simulink model "PatchedConic"  (R2022b)
settings: Solver=ode4  StartTime=0.0  StopTime=simTime  FixedStep=dt  RelTol=1e-3
values from neighbouring files (symbols this model uses):
  dv1 = [0,0.730140014317,0]    [main.m]
  lunar_distance = 388000    [main.m]
  lunar_w = [0,0,2*pi / (27*24*3600)]    [main.m]
  lunar_wn = 2*pi / (27*24*3600)    (= 2.6934093395e-06)    [main.m]
  mu_earth = 398600    [main.m]
  mu_lunar = 4911.3    [main.m]
  r0_inj = [lunar_distance - lunar_SOI ,0,0]    [main.m]
  r0_trans = [ - R_earth - altitude , 0 , 0]    [main.m]
  T_inj = 167185    [main.m]
  T_trans = pi * sqrt( a_trans ^3 / mu_earth )    [main.m]
  v0_inj = [ 0 , sqrt( mu_earth * ( 2 / (lunar_distance - lunar_SOI ) - 1 / a_trans ) ) , 0]    [main.m]
  v0_trans = [ 0 , -sqrt( mu_earth * ( 2 / norm(r0_trans) - 1 / a_trans ) ) , 0 ]    [main.m]
  v_need = sqrt ( mu_lunar / ( R_lunar + Rmission ) )    [main.m]
libraries: matrix_library x1
settings Model: Creator=dongmin  LastModifiedBy=dongmin

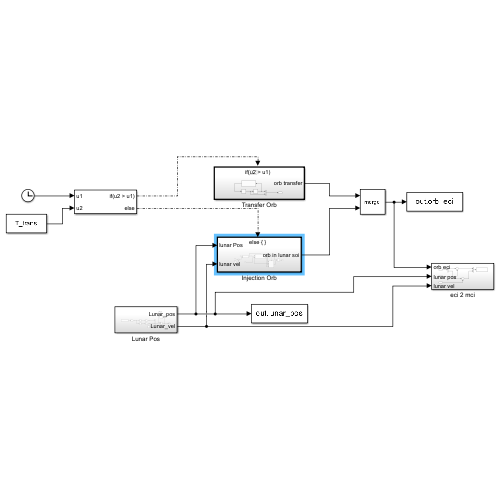
[thumbnail: Simulink's stored preview of the top-level diagram]
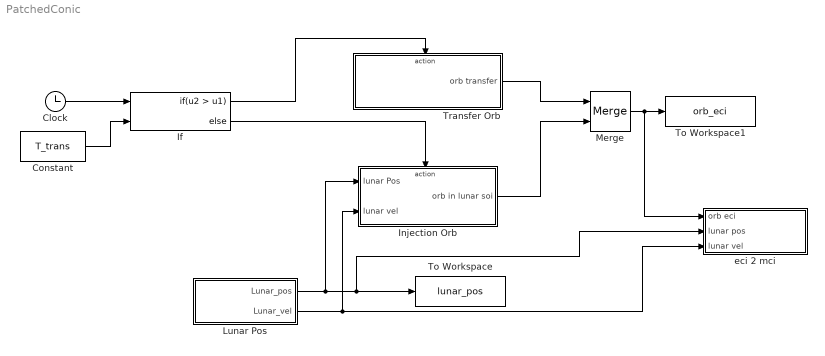
== system PatchedConic ==
  Clock : Clock
  Constant : Constant  Value=T_trans
  If : If  NumInputs=2  IfExpression=u2 > u1
  Injection Orb : Subsystem  TreatAsAtomicUnit=on
  Lunar Pos : Subsystem
  Merge : Merge
  To Workspace : ToWorkspace  VariableName=lunar_pos  SaveFormat=Timeseries  SampleTime=-1
  To Workspace1 : ToWorkspace  VariableName=orb_eci  SaveFormat=Timeseries  SampleTime=-1
  Transfer Orb : Subsystem  TreatAsAtomicUnit=on
  eci 2 mci : Subsystem
  wires:
  Clock/1 -> If/1
  Constant/1 -> If/2
  If/1 -> Transfer Orb/Action
  If/2 -> Injection Orb/Action
  Lunar Pos/1(Lunar_pos) -> Injection Orb/1(lunar Pos), eci 2 mci/2(lunar pos), To Workspace/1
  Transfer Orb/1(orb transfer) -> Merge/1
  Injection Orb/1(orb in lunar soi) -> Merge/2
  Merge/1 -> eci 2 mci/1(orb eci), To Workspace1/1
  Lunar Pos/2(Lunar_vel) -> Injection Orb/2(lunar vel), eci 2 mci/3(lunar vel)

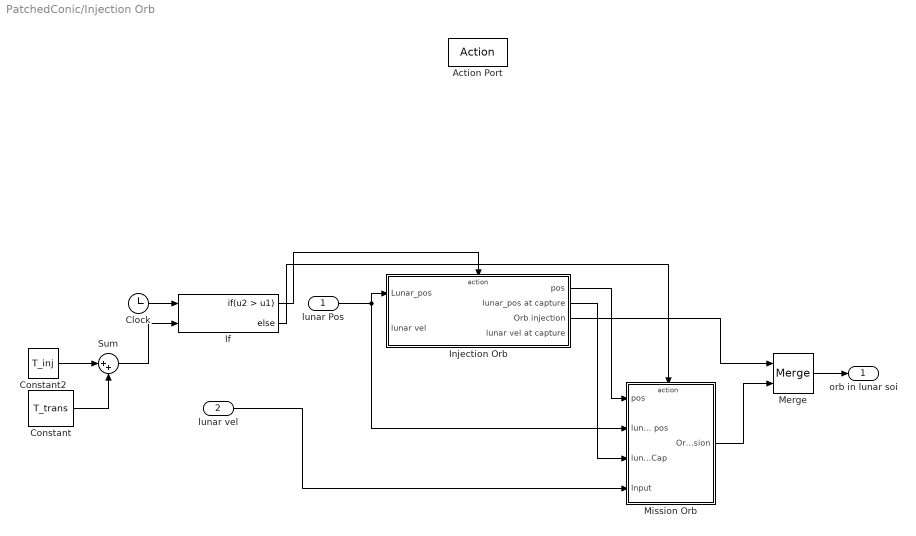
== system PatchedConic/Injection Orb ==
  lunar Pos : Inport
  lunar vel : Inport  Port=2
  Action Port : ActionPort  ActionPortLabel=else
  Clock : Clock
  Constant : Constant  Value=T_trans
  Constant2 : Constant  Value=T_inj
  If : If  NumInputs=2  IfExpression=u2 > u1
  Injection Orb : Subsystem  TreatAsAtomicUnit=on
  Merge : Merge
  Mission Orb : Subsystem  TreatAsAtomicUnit=on
  Sum : Sum  Inputs=|++
  orb in lunar soi : Outport
  wires:
  Clock/1 -> If/1
  Constant2/1 -> Sum/1
  If/1 -> Injection Orb/Action
  lunar Pos/1 -> Mission Orb/2(lunar pos), Injection Orb/1(Lunar_pos)
  If/2 -> Mission Orb/Action
  Injection Orb/1(pos) -> Mission Orb/1(pos)
  Constant/1 -> Sum/2
  Sum/1 -> If/2
  Injection Orb/2(lunar_pos at capture) -> Mission Orb/3(lunar_posAtCap)
  Injection Orb/3(Orb injection) -> Merge/1
  Mission Orb/1(Orb_mission) -> Merge/2
  Merge/1 -> orb in lunar soi/1
  lunar vel/1 -> Mission Orb/4(Input)

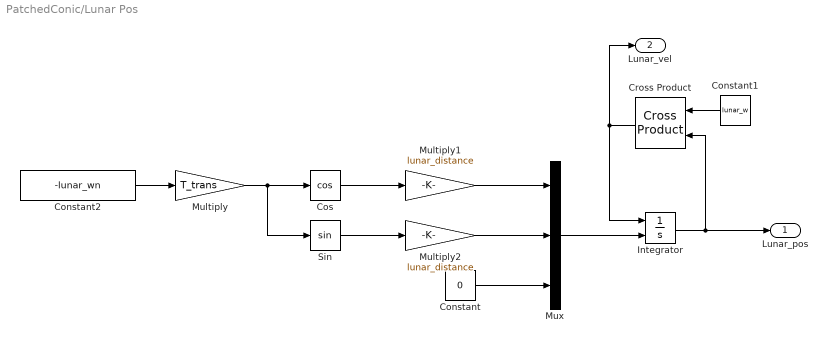
== system PatchedConic/Lunar Pos ==
  Constant : Constant  Value=0
  Constant1 : Constant  Value=lunar_w
  Constant2 : Constant  Value=-lunar_wn
  Cos : Trigonometry  Operator=cos
  Cross Product : matrix_library/Cross Product
  Integrator : Integrator  InitialConditionSource=external
  Multiply : Gain  Gain=T_trans
  Multiply1 : Gain  Gain=lunar_distance
  Multiply2 : Gain  Gain=lunar_distance
  Mux : Mux  Inputs=3
  Sin : Trigonometry
  Lunar_pos : Outport
  Lunar_vel : Outport  Port=2
  wires:
  Constant2/1 -> Multiply/1
  Multiply/1 -> Sin/1, Cos/1
  Cos/1 -> Multiply1/1
  Sin/1 -> Multiply2/1
  Multiply1/1 -> Mux/1
  Multiply2/1 -> Mux/2
  Constant/1 -> Mux/3
  Integrator/1 -> Cross Product/2, Lunar_pos/1
  Constant1/1 -> Cross Product/1
  Cross Product/1 -> Integrator/1, Lunar_vel/1
  Mux/1 -> Integrator/2

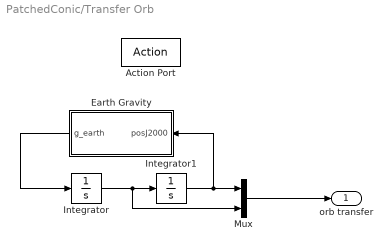
== system PatchedConic/Transfer Orb ==
  Action Port : ActionPort  ActionPortLabel=if(u2 > u1)
  Earth Gravity : Subsystem
  Integrator : Integrator  InitialCondition=v0_trans
  Integrator1 : Integrator  InitialCondition=r0_trans
  Mux : Mux  Inputs=2
  orb transfer : Outport
  wires:
  Mux/1 -> orb transfer/1
  Integrator1/1 -> Earth Gravity/1(posJ2000), Mux/1
  Integrator/1 -> Mux/2, Integrator1/1
  Earth Gravity/1(g_earth) -> Integrator/1

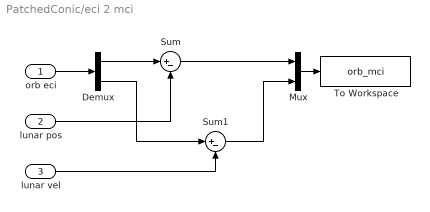
== system PatchedConic/eci 2 mci ==
  orb eci : Inport
  lunar pos : Inport  Port=2
  lunar vel : Inport  Port=3
  Demux : Demux  Outputs=2
  Mux : Mux  Inputs=2
  Sum : Sum  Inputs=|+-
  Sum1 : Sum  Inputs=|+-
  To Workspace : ToWorkspace  VariableName=orb_mci  SaveFormat=Timeseries  SampleTime=-1
  wires:
  orb eci/1 -> Demux/1
  Demux/1 -> Sum/1
  lunar pos/1 -> Sum/2
  Sum/1 -> Mux/1
  Demux/2 -> Sum1/1
  lunar vel/1 -> Sum1/2
  Sum1/1 -> Mux/2
  Mux/1 -> To Workspace/1

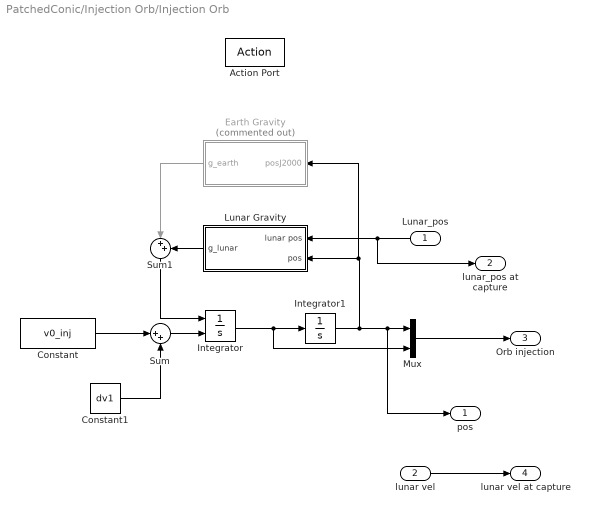
== system PatchedConic/Injection Orb/Injection Orb ==
  Lunar_pos : Inport
  lunar vel : Inport  Port=2
  Action Port : ActionPort  ActionPortLabel=if(u2 > u1)
  Constant : Constant  Value=v0_inj
  Constant1 : Constant  Value=dv1
  Earth Gravity : Subsystem  Commented=on
  Integrator : Integrator  InitialConditionSource=external  InitialCondition=v0_inj
  Integrator1 : Integrator  InitialCondition=r0_inj
  Lunar Gravity : Subsystem
  Mux : Mux  Inputs=2
  Sum : Sum  Inputs=|++
  Sum1 : Sum  Inputs=|++
  pos : Outport
  lunar_pos at capture : Outport  Port=2
  Orb injection : Outport  Port=3
  lunar vel at capture : Outport  Port=4
  wires:
  Constant1/1 -> Sum/2
  Lunar_pos/1 -> lunar_pos at capture/1, Lunar Gravity/1(lunar pos)
  Constant/1 -> Sum/1
  Lunar Gravity/1(g_lunar) -> Sum1/2
  Integrator1/1 -> pos/1, Mux/1, Earth Gravity/1(posJ2000), Lunar Gravity/2(pos)
  Integrator/1 -> Mux/2, Integrator1/1
  Sum/1 -> Integrator/2
  Mux/1 -> Orb injection/1
  lunar vel/1 -> lunar vel at capture/1
  Earth Gravity/1(g_earth) -> Sum1/1
  Sum1/1 -> Integrator/1

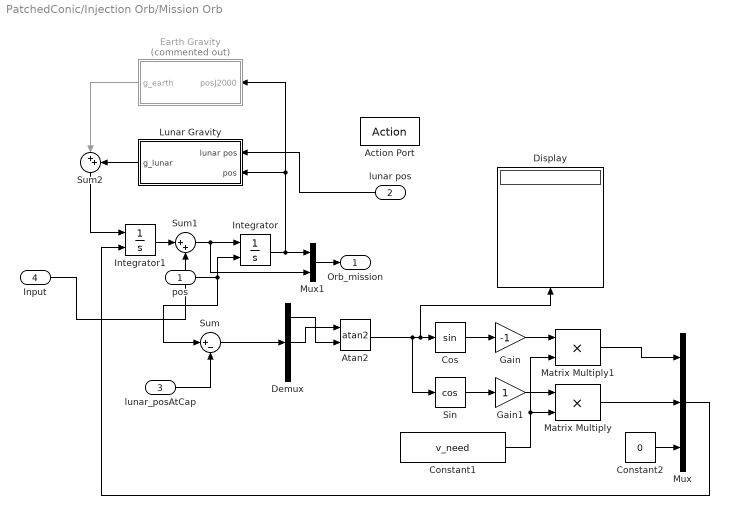
== system PatchedConic/Injection Orb/Mission Orb ==
  pos : Inport
  lunar pos : Inport  Port=2
  lunar_posAtCap : Inport  Port=3
  Input : Inport  Port=4
  Action Port : ActionPort  ActionPortLabel=else
  Atan2 : Trigonometry  Operator=atan2
  Constant1 : Constant  Value=v_need
  Constant2 : Constant  Value=0
  Cos : Trigonometry
  Demux : Demux  Outputs=3
  Display : Display
  Earth Gravity : Subsystem  Commented=on
  Gain : Gain  Gain=-1
  Gain1 : Gain
  Integrator : Integrator  InitialConditionSource=external
  Integrator1 : Integrator  InitialConditionSource=external
  Lunar Gravity : Subsystem
  Matrix Multiply : Product
  Matrix Multiply1 : Product
  Mux : Mux  Inputs=3
  Mux1 : Mux  Inputs=2
  Sin : Trigonometry  Operator=cos
  Sum : Sum  Inputs=|+-
  Sum1 : Sum  Inputs=|++
  Sum2 : Sum  Inputs=|++
  Orb_mission : Outport
  wires:
  pos/1 -> Integrator/2, Sum/1
  Integrator/1 -> Mux1/1, Earth Gravity/1(posJ2000), Lunar Gravity/2(pos)
  lunar pos/1 -> Lunar Gravity/1(lunar pos)
  Lunar Gravity/1(g_lunar) -> Sum2/2
  lunar_posAtCap/1 -> Sum/2
  Sum/1 -> Demux/1
  Demux/1 -> Atan2/2
  Atan2/1 -> Display/1, Cos/1, Sin/1
  Constant1/1 -> Matrix Multiply1/2, Matrix Multiply/2
  Cos/1 -> Gain/1
  Matrix Multiply/1 -> Mux/2
  Sin/1 -> Gain1/1
  Matrix Multiply1/1 -> Mux/1
  Gain/1 -> Matrix Multiply1/1
  Constant2/1 -> Mux/3
  Demux/2 -> Atan2/1
  Mux1/1 -> Orb_mission/1
  Mux/1 -> Integrator1/2
  Gain1/1 -> Matrix Multiply/1
  Integrator1/1 -> Sum1/1
  Sum1/1 -> Mux1/2, Integrator/1
  Earth Gravity/1(g_earth) -> Sum2/1
  Sum2/1 -> Integrator1/1
  Input/1 -> Sum1/2

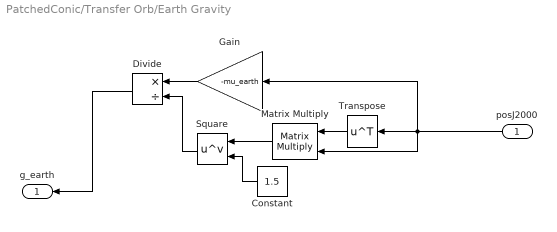
== system PatchedConic/Transfer Orb/Earth Gravity ==
  posJ2000 : Inport
  Constant : Constant  Value=1.5
  Divide : Product  Inputs=*/
  Gain : Gain  Gain=-mu_earth
  Matrix Multiply : Product  Multiplication=Matrix(*)
  Square : Math  Operator=pow
  Transpose : Math  Operator=transpose
  g_earth : Outport
  wires:
  Square/1 -> Divide/2
  Matrix Multiply/1 -> Square/1
  Divide/1 -> g_earth/1
  Gain/1 -> Divide/1
  Transpose/1 -> Matrix Multiply/1
  Constant/1 -> Square/2
  posJ2000/1 -> Transpose/1, Gain/1, Matrix Multiply/2

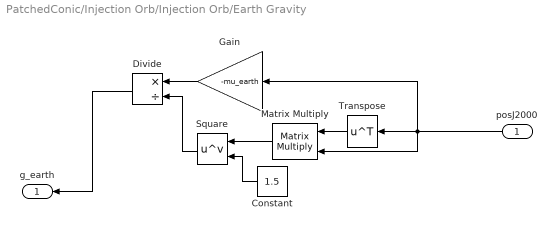
== system PatchedConic/Injection Orb/Injection Orb/Earth Gravity ==
  posJ2000 : Inport
  Constant : Constant  Value=1.5
  Divide : Product  Inputs=*/
  Gain : Gain  Gain=-mu_earth
  Matrix Multiply : Product  Multiplication=Matrix(*)
  Square : Math  Operator=pow
  Transpose : Math  Operator=transpose
  g_earth : Outport
  wires:
  Square/1 -> Divide/2
  Matrix Multiply/1 -> Square/1
  Divide/1 -> g_earth/1
  Gain/1 -> Divide/1
  Transpose/1 -> Matrix Multiply/1
  Constant/1 -> Square/2
  posJ2000/1 -> Transpose/1, Gain/1, Matrix Multiply/2

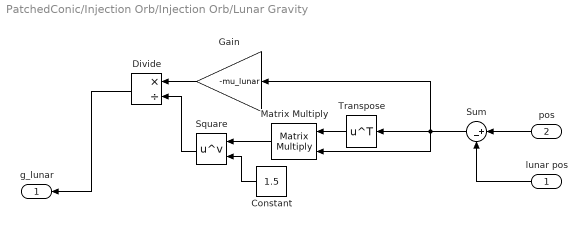
== system PatchedConic/Injection Orb/Injection Orb/Lunar Gravity ==
  lunar pos : Inport
  pos : Inport  Port=2
  Constant : Constant  Value=1.5
  Divide : Product  Inputs=*/
  Gain : Gain  Gain=-mu_lunar
  Matrix Multiply : Product  Multiplication=Matrix(*)
  Square : Math  Operator=pow
  Sum : Sum  Inputs=|+-
  Transpose : Math  Operator=transpose
  g_lunar : Outport
  wires:
  Constant/1 -> Square/2
  Transpose/1 -> Matrix Multiply/1
  Square/1 -> Divide/2
  Divide/1 -> g_lunar/1
  Gain/1 -> Divide/1
  Matrix Multiply/1 -> Square/1
  Sum/1 -> Gain/1, Matrix Multiply/2, Transpose/1
  pos/1 -> Sum/1
  lunar pos/1 -> Sum/2

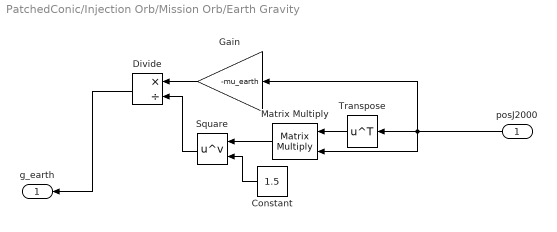
== system PatchedConic/Injection Orb/Mission Orb/Earth Gravity ==
  posJ2000 : Inport
  Constant : Constant  Value=1.5
  Divide : Product  Inputs=*/
  Gain : Gain  Gain=-mu_earth
  Matrix Multiply : Product  Multiplication=Matrix(*)
  Square : Math  Operator=pow
  Transpose : Math  Operator=transpose
  g_earth : Outport
  wires:
  Square/1 -> Divide/2
  Matrix Multiply/1 -> Square/1
  Divide/1 -> g_earth/1
  Gain/1 -> Divide/1
  Transpose/1 -> Matrix Multiply/1
  Constant/1 -> Square/2
  posJ2000/1 -> Transpose/1, Gain/1, Matrix Multiply/2

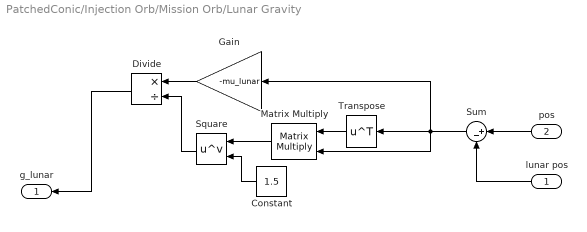
== system PatchedConic/Injection Orb/Mission Orb/Lunar Gravity ==
  lunar pos : Inport
  pos : Inport  Port=2
  Constant : Constant  Value=1.5
  Divide : Product  Inputs=*/
  Gain : Gain  Gain=-mu_lunar
  Matrix Multiply : Product  Multiplication=Matrix(*)
  Square : Math  Operator=pow
  Sum : Sum  Inputs=|+-
  Transpose : Math  Operator=transpose
  g_lunar : Outport
  wires:
  Sum/1 -> Gain/1, Matrix Multiply/2, Transpose/1
  pos/1 -> Sum/1
  lunar pos/1 -> Sum/2
  Square/1 -> Divide/2
  Constant/1 -> Square/2
  Gain/1 -> Divide/1
  Matrix Multiply/1 -> Square/1
  Divide/1 -> g_lunar/1
  Transpose/1 -> Matrix Multiply/1
